simulink model "antbotII_trajectory_planning_leg1"  (R2017b)
settings: Solver=VariableStepAuto  StartTime=0.0  StopTime=2.0  RelTol=1e-3
undefined symbols (not defined in the file or in its folder): sigbuilder_block
libraries: simulink x1
settings Model: Creator=nekou  LastModifiedBy=nekou

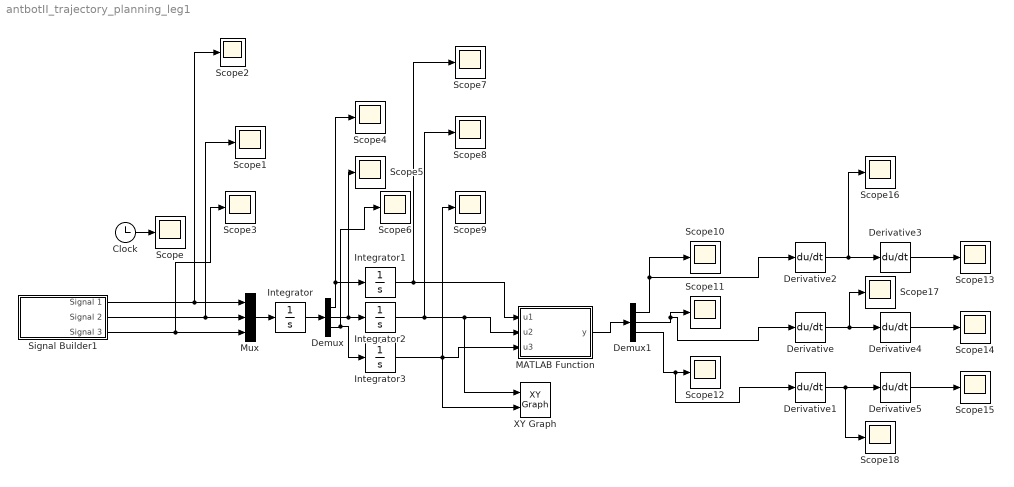
== system antbotII_trajectory_planning_leg1 ==
  Clock : Clock
  Demux : Demux  Outputs=3
  Demux1 : Demux  Outputs=3
  Derivative{,1..5} (6 alike) : Derivative
  Integrator : Integrator
  Integrator1 : Integrator  InitialCondition=111.310
  Integrator2 : Integrator  InitialCondition=192.794
  Integrator3 : Integrator  InitialCondition=-148.031
  MATLAB Function : MATLAB Function  TreatAsAtomicUnit=on
  Mux : Mux  Inputs=3
  Scope{,1..18} (19 alike) : Scope
  Signal Builder1 : Subsystem  Tag=STV Subsys  LoadFcn=sigbuilder_block('load');  StartFcn=sigbuilder_block('start');  StopFcn=sigbuilder_block('stop');  ClipboardFcn=sigbuilder_block('clipboard');  mask(Sigbuilder block){tuvar=[0:10]}
      mask help: Simulink:masks:SigbuilderBlock_MD
      mask init:
      | if ~strcmp(get_param(bdroot(gcbh),'SimulationStatus'),'stopped') tuvar = sigbuilder_block('maskInit'); end
      settings: CopyFcn=sigbuilder_block('copy');  DeleteFcn=sigbuilder_block('delete');  ModelCloseFcn=sigbuilder_block('modelClose');  PreSaveFcn=sigbuilder_block('preSave');  PauseFcn=sigbuilder_block('pause');  ContinueFcn=sigbuilder_block('continue');  NameChangeFcn=sigbuilder_block('namechange');  OpenFcn=sigbuilder_block('open',[6 6 1012.5 506.25 ]);  CloseFcn=sigbuilder_block('close');
      mask Display: plot(0, 0, 100, 100,[2, 2, 32, 32, 2], [68, 8, 8, 68, 68],[32, 2], [38, 38], [32, 19, 2],[53, 60, 44], [32, 17, 17, 2],[16, 16, 31, 31]);txt = getActiveGroup(gcbh);text(2, 100, txt,'verticalAlignment', 'top');
  XY Graph : simulink/Sinks/XY Graph  xmin=200  xmax=400  ymin=-150  ymax=-40  st=-1
  wires:
  Clock/1 -> Scope/1
  Signal Builder1/1(Signal 1) -> Mux/1, Scope2/1
  Mux/1 -> Integrator/1
  Integrator/1 -> Demux/1
  Demux/2 -> Integrator2/1, Scope5/1
  Demux/1 -> Integrator1/1, Scope4/1
  Demux/3 -> Integrator3/1, Scope6/1
  Integrator1/1 -> MATLAB Function/1(u1), Scope7/1
  Integrator2/1 -> Scope8/1, XY Graph/1, MATLAB Function/2(u2)
  Integrator3/1 -> XY Graph/2, Scope9/1, MATLAB Function/3(u3)
  MATLAB Function/1(y) -> Demux1/1
  Demux1/1 -> Derivative2/1, Scope10/1
  Demux1/2 -> Derivative/1, Scope11/1
  Demux1/3 -> Derivative1/1, Scope12/1
  Derivative/1 -> Scope17/1, Derivative4/1
  Derivative2/1 -> Scope16/1, Derivative3/1
  Derivative1/1 -> Scope18/1, Derivative5/1
  Derivative3/1 -> Scope13/1
  Derivative4/1 -> Scope14/1
  Derivative5/1 -> Scope15/1
  Signal Builder1/2(Signal 2) -> Mux/2, Scope1/1
  Signal Builder1/3(Signal 3) -> Scope3/1, Mux/3

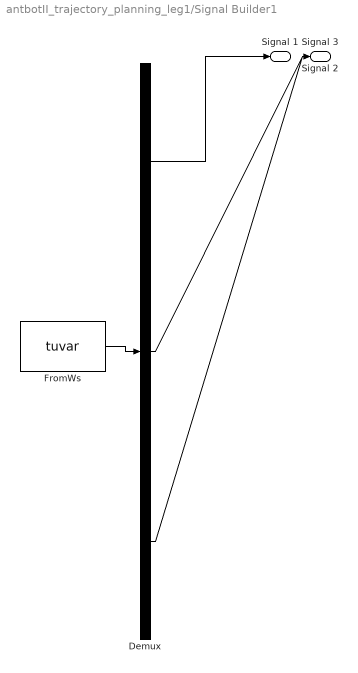
== system antbotII_trajectory_planning_leg1/Signal Builder1 ==
  Demux : Demux  Tag=STV Demux  Outputs=3
  FromWs : FromWorkspace  Tag=STV FromWs  VariableName=tuvar  SampleTime=0
      SigBuilderData=|
      | common.afterFinalStr = 'Extrapolate'
      | common.sampleTime = 0
      | dataSet.timeRange = [0 10]
      | dataSet.name = 'Group 1'
      | sbobj.Groups.Name = 'Group 1'
      | sbobj.Groups.Signals(1).Name = 'Signal 1'
      | sbobj.Groups.Signals(1).XData = [0 10]
      | sbobj.Groups.Signals(1).YData = [0 0]
      | sbobj.Groups.Signals(2).Name = 'Signal 2'
      | sbobj.Groups.Signals(2).XData = [0 10]
      | sbobj.Groups.Signals(2).YData = [75 -675]
      | sbobj.Groups.Signals(3).Name = 'Signal 3'
      | sbobj.Groups.Signals(3).XData = [0 1 2 10]
      | sbobj.Groups.Signals(3).YData = [150 -150 150 150]
  Signal 1 : Outport  Tag=STV Outport
  Signal 2 : Outport  Tag=STV Outport  Port=2
  Signal 3 : Outport  Tag=STV Outport  Port=3
  wires:
  Demux/1 -> Signal 1/1
  FromWs/1 -> Demux/1
  Demux/2 -> Signal 2/1
  Demux/3 -> Signal 3/1

== matlab function antbotII_trajectory_planning_leg1/MATLAB Function ==
  data: u1 input; y output; u2 input; u3 input
function y = fcn(u1,u2,u3)
xprime1 = u1;
yprime1 = u2;
zprime1 = u3+17;
% xprime1 = 111.310; %213.6188;
% yprime1 = 192.794; %284.3948;
% zprime1 = -148.031+17; %-155.7892+15.68;
xoffset1 = 71.6; %60.827;
X1 = xprime1-xoffset1;
yoffset1 = 120.96;%131.38;
Y1 = yprime1-yoffset1;
zoffset1 = 17.00;
Z1 = zprime1-zoffset1;
L1 = 66.5;
L2 = 92.17;
L3 = 193.66;
offsetang = pi/3;
theta11 = (atan2(Y1, X1)-offsetang);
newx = cos(-1*offsetang)*X1 - sin(-1*offsetang)*Y1;
newy = sin(-1*offsetang)*X1 + cos(-1*offsetang)*Y1;
x1 = cos(theta11)*(newx) + sin(theta11)*(newy) - L1;
y1 = sin(theta11)*(newx) - cos(theta11)*(newy);
s1 = sqrt(x1^2 + zprime1^2);
t13 = pi -acos(( - s1^2 + L2^2 + L3^2)/(2*L2*L3));
theta13 = t13 - 73.27 *pi/180;
theta12 = - atan2(zprime1, x1) - atan2(L3*sin(t13), L2 + L3*cos(t13)) + (20)*pi/180;
theta11indegs1 = (theta11+pi)*180/pi;
theta12indegs1 = (-theta12+pi)*180/pi;
theta13indegs1 = (-theta13+pi)*180/pi;
out = [theta11indegs1*4096/360;theta12indegs1*4096/360;theta13indegs1*4096/360];
y = out
